simulink model "ULA_4ant_sim2a"  (R2018b)
settings: Solver=VariableStepAuto  StartTime=0.0  StopTime=0.1  RelTol=1e-3
values from neighbouring files (symbols this model uses):
  d = wl/2    [BS1.m]    (also in BS2.m; LU1.m = 0.172691508065; QR2M.m = 0.172691508065; QR3_theta.m = 0.172691508065)
  M = 4    [BS1.m]    (also in BS2.m; LU1.m; QR2M.m; QR3_theta.m)
undefined symbols (not defined in the file or in its folder): phased, physconst
libraries: dspsrcs4 x3, phasedtxrxlib x2
settings Model: Creator=Wei S  LastModifiedBy=Wei S

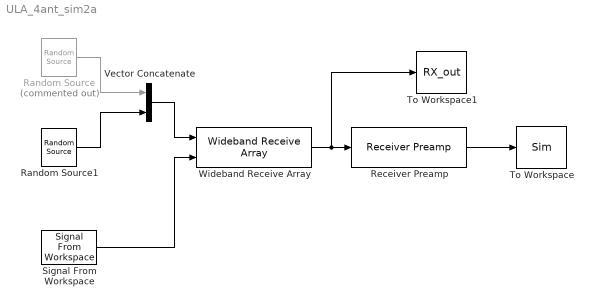
== system ULA_4ant_sim2a ==
  Random Source : dspsrcs4/Random Source  Commented=on  SrcType=Gaussian  NormMethod=Ziggurat  CltLength=12  MinVal=0  MaxVal=1  MeanVal=0  VarVal=100  RepMode=Repeatable  rawSeed=1  IsInherit=off  SampMode=Discrete  SampTime=1/1000  SampFrame=300  DataType=Double  OutComplex=Real  OutputFrames=off
  Random Source1 : dspsrcs4/Random Source  SrcType=Gaussian  NormMethod=Ziggurat  CltLength=12  MinVal=0  MaxVal=1  MeanVal=0  VarVal=100  RepMode=Repeatable  rawSeed=1  IsInherit=off  SampMode=Discrete  SampTime=1/1000  SampFrame=300  DataType=Double  OutComplex=Real  OutputFrames=off
  Receiver Preamp : phasedtxrxlib/Receiver Preamp  Gain=0  LossFactor=0  NoiseMethod=Noise power  NoiseFigure=NF  ReferenceTemperature=290  SampleRateFromInputCheckbox=on  SampleRate=1e6  NoisePower=0.1  EnableInputPort=off  PhaseNoiseInputPort=off  SeedSource=Property  Seed=randi(65535,1)  SimulateUsing=Interpreted execution
      settings: SourceProductName=Phased Array System Toolbox  SourceProductBaseCode=AR
  Signal From Workspace : dspsrcs4/Signal From Workspace  X=Ang  Ts=0.3  nsamps=1  OutputAfterFinalValue=Setting to zero  ignoreOrWarnInputAndFrameLengths=off  OutputFrames=off
  To Workspace : ToWorkspace  VariableName=Sim  SampleTime=-1
      settings: Save2DSignal=2-D array (concatenate along first dimension)
  To Workspace1 : ToWorkspace  VariableName=RX_out  SampleTime=-1
      settings: Save2DSignal=2-D array (concatenate along first dimension)
  Vector Concatenate : Concatenate
  Wideband Receive Array : phasedtxrxlib/Wideband Receive Array  PropagationSpeed=physconst( 'LightSpeed' )  SampleRateFromInputCheckbox=on  SampleRate=1e6  ModulatedInput=on  CarrierFrequency=8.68e8  NumSubbands=1  Wavefront=Plane  SensorGainMeasure=dB  Polarization=None  WeightsInputPort=off  SimulateUsing=Interpreted execution  Sensor=phased.ULA('Element',phased.IsotropicAntennaElement(),'NumElements',M,'ElementSpacing',d)
      settings: SourceProductName=Phased Array System Toolbox  SourceProductBaseCode=AR
  wires:
  Vector Concatenate/1 -> Wideband Receive Array/1
  Random Source1/1 -> Vector Concatenate/2
  Signal From Workspace/1 -> Wideband Receive Array/2
  Receiver Preamp/1 -> To Workspace/1
  Random Source/1 -> Vector Concatenate/1
  Wideband Receive Array/1 -> To Workspace1/1, Receiver Preamp/1
